simulink model "Btech_sys1"  (R2023b)
settings: Solver=VariableStepAuto  StartTime=0.0  StopTime=50  RelTol=1e-3
values from neighbouring files (symbols this model uses):
  Kd1 = x(1,3)    [fopid_pso.m]    (also in main_SHO_FOPID.m = Sea_horses(i,2); main_SHO_FOPTID.m = Sea_horses(i,2); main_SHO_PID.m = Sea_horses(i,2); pso.m)
  Kd2 = x(1,7)    [fopid_pso.m]    (also in main_SHO_FOPID.m = Sea_horses(i,5); main_SHO_FOPTID.m = Sea_horses(i,6); main_SHO_PID.m = Sea_horses(i,5); pso.m)
  Ki1 = x(1,2)    [fopid_pso.m]    (also in main_SHO_FOPID.m = Sea_horses(i,3); main_SHO_FOPTID.m = Sea_horses(i,3); main_SHO_PID.m = Sea_horses(i,3); pso.m)
  Ki2 = x(1,6)    [fopid_pso.m]    (also in main_SHO_FOPID.m = Sea_horses(i,6); main_SHO_FOPTID.m = Sea_horses(i,7); main_SHO_PID.m = Sea_horses(i,6); pso.m)
  Kp1 = x(1,1)    [fopid_pso.m]    (also in main_SHO_FOPID.m = Sea_horses(i,1); main_SHO_FOPTID.m = Sea_horses(i,1); main_SHO_PID.m = Sea_horses(i,1); pso.m)
  Kp2 = x(1,5)    [fopid_pso.m]    (also in main_SHO_FOPID.m = Sea_horses(i,4); main_SHO_FOPTID.m = Sea_horses(i,5); main_SHO_PID.m = Sea_horses(i,4); pso.m)
  Kt1 = Sea_horses(i,4)    [main_SHO_FOPTID.m]
  Kt2 = Sea_horses(i,8)    [main_SHO_FOPTID.m]
  N1 = Sea_horses(i,15)    [main_SHO_FOPTID.m]    (also in main_SHO_PID.m = Sea_horses(i,7); pso.m = x(1,4))
  N2 = Sea_horses(i,16)    [main_SHO_FOPTID.m]    (also in main_SHO_PID.m = Sea_horses(i,8); pso.m = x(1,8))
libraries: fod x10, slpidlib x2
settings Model: Creator=V.Abhijith  LastModifiedBy=V.Abhijith

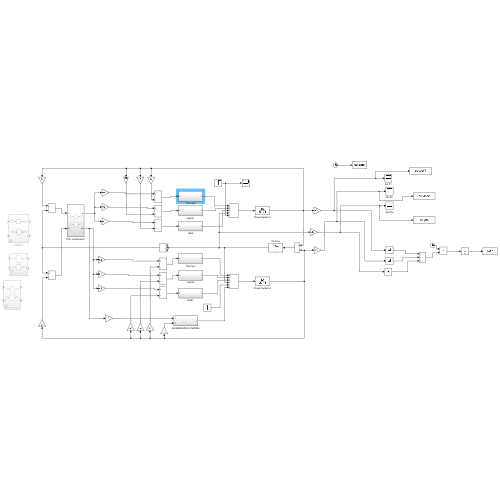
[thumbnail: Simulink's stored preview of the top-level diagram]
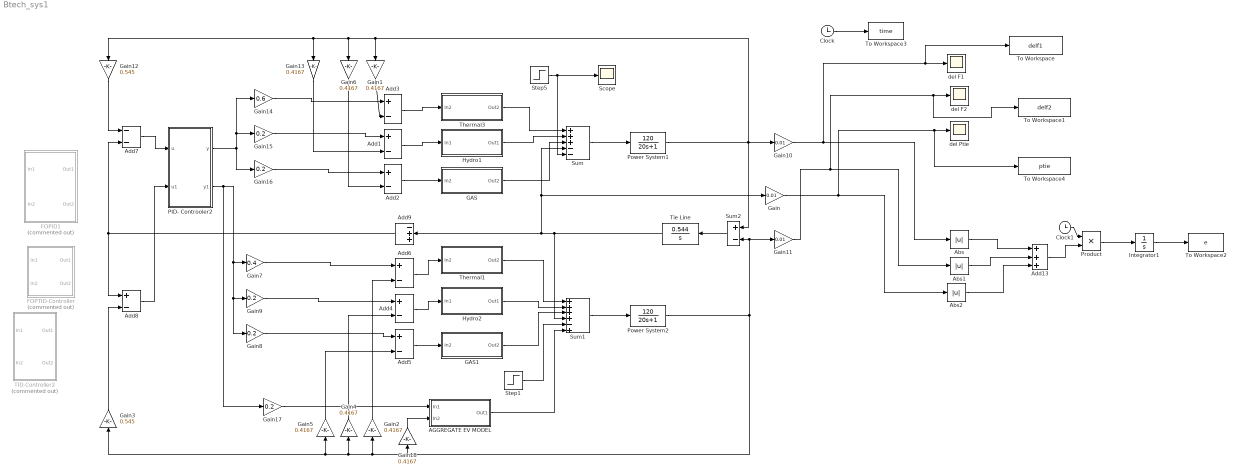
== system Btech_sys1 ==
  AGGREGATE EV MODEL : Subsystem
  Abs : Abs  SaturateOnIntegerOverflow=off
  Abs1 : Abs  SaturateOnIntegerOverflow=off
  Abs2 : Abs  SaturateOnIntegerOverflow=off
  Add{1..6,8} (7 alike) : Sum  Inputs=+-
  Add13 : Sum  Inputs=+++
  Add7 : Sum  Inputs=--
  Add9 : Sum  Inputs=-++
  Clock : Clock
  Clock1 : Clock
  FOPID1 : Subsystem  Commented=on
  FOPTID-Controller : Subsystem  Commented=on
  GAS : Subsystem
  GAS1 : Subsystem
  Gain : Gain  Gain=0.01
  Gain{1..2,4..6,13,18} (7 alike) : Gain  Gain=0.4167
  Gain10 : Gain  Gain=0.01
  Gain11 : Gain  Gain=0.01
  Gain12 : Gain  Gain=0.545
  Gain14 : Gain  Gain=0.6
  Gain{8..9,15..17} (5 alike) : Gain  Gain=0.2
  Gain3 : Gain  Gain=0.545
  Gain7 : Gain  Gain=0.4
  Hydro1 : Subsystem
  Hydro2 : Subsystem
  Integrator1 : Integrator
  PID- Controoler2 : Subsystem
  Power System1 : TransferFcn  Numerator=[120]  Denominator=[20 1]
  Power System2 : TransferFcn  Numerator=[120]  Denominator=[20 1]
  Product : Product
  Scope : Scope
  Step1 : Step  Time=0  After=0.03  SampleTime=0  ZeroCross=off
  Step5 : Step  Time=0  After=0.03  SampleTime=0  ZeroCross=off
  Sum : Sum  Inputs=+++--
  Sum1 : Sum  Inputs=++++-+
  Sum2 : Sum  Inputs=+-
  TID-Controller2 : Subsystem  Commented=on
  Thermal1 : Subsystem
  Thermal3 : Subsystem
  Tie Line : TransferFcn  Numerator=[0.544]  Denominator=[1 0]
  To Workspace : ToWorkspace  VariableName=delf1  SaveFormat=Timeseries  SampleTime=-1
  To Workspace1 : ToWorkspace  VariableName=delf2  SaveFormat=Timeseries  SampleTime=-1
  To Workspace2 : ToWorkspace  VariableName=e  SampleTime=-1
      settings: MaxDataPoints=1
  To Workspace3 : ToWorkspace  VariableName=time  SampleTime=-1
  To Workspace4 : ToWorkspace  VariableName=ptie  SaveFormat=Timeseries  SampleTime=-1
  del F1 : Scope
  del F2 : Scope
  del Ptie : Scope
  wires:
  Add8/1 -> PID- Controoler2/2(u1)
  Abs1/1 -> Add13/2
  Add4/1 -> Hydro2/1(In1)
  Step1/1 -> Sum1/5
  Tie Line/1 -> Add9/2, Gain/1, Sum/4, Sum1/4
  Abs2/1 -> Add13/3
  Add2/1 -> GAS/1(In2)
  Integrator1/1 -> To Workspace2/1
  Clock1/1 -> Product/1
  GAS1/1(Out2) -> Sum1/3
  PID- Controoler2/1(y) -> Gain16/1, Gain15/1, Gain14/1
  GAS/1(Out2) -> Sum/3
  Gain13/1 -> Add1/2
  Power System1/1 -> Gain10/1, Sum2/1, Gain12/1, Gain13/1, Gain6/1, Gain1/1
  Gain16/1 -> Add2/1
  Gain8/1 -> Add5/1
  Hydro2/1(Out1) -> Sum1/2
  Gain9/1 -> Add4/1
  Add1/1 -> Hydro1/1(In1)
  Hydro1/1(Out1) -> Sum/2
  Gain12/1 -> Add7/1
  Gain7/1 -> Add6/1
  Gain6/1 -> Add2/2
  Sum1/1 -> Power System2/1
  Sum/1 -> Power System1/1
  Gain5/1 -> Add5/2
  Add5/1 -> GAS1/1(In2)
  Sum2/1 -> Tie Line/1
  Thermal1/1(Out2) -> Sum1/1
  Product/1 -> Integrator1/1
  Gain3/1 -> Add8/2
  Power System2/1 -> Gain11/1, Sum2/2, Gain18/1, Gain3/1, Gain5/1, Gain4/1, Gain2/1
  Clock/1 -> To Workspace3/1
  Add9/1 -> Add8/1, Add7/2
  Step5/1 -> Sum/5, Scope/1
  Gain1/1 -> Add3/2
  Add6/1 -> Thermal1/1(In2)
  Gain4/1 -> Add4/2
  Abs/1 -> Add13/1
  Add7/1 -> PID- Controoler2/1(u)
  Gain2/1 -> Add6/2
  Gain15/1 -> Add1/1
  Gain14/1 -> Add3/1
  PID- Controoler2/2(y1) -> Gain17/1, Gain8/1, Gain9/1, Gain7/1
  Add13/1 -> Product/2
  Add3/1 -> Thermal3/1(In2)
  Thermal3/1(Out2) -> Sum/1
  AGGREGATE EV MODEL/1(Out1) -> Sum1/6
  Gain10/1 -> To Workspace/1, del F1/1, Abs/1
  Gain/1 -> To Workspace4/1, del Ptie/1, Abs2/1
  Gain11/1 -> To Workspace1/1, del F2/1, Abs1/1
  Gain17/1 -> AGGREGATE EV MODEL/1(In1)
  Gain18/1 -> AGGREGATE EV MODEL/2(In2)

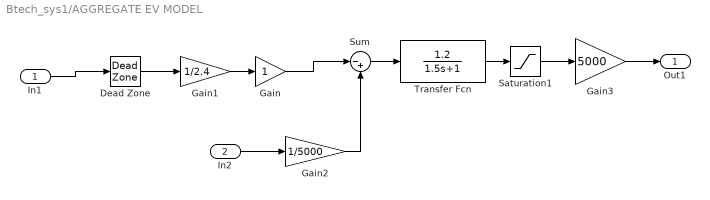
== system Btech_sys1/AGGREGATE EV MODEL ==
  In1 : Inport
  In2 : Inport  Port=2
  Dead Zone : DeadZone  LowerValue=-0.01  UpperValue=0.01
  Gain : Gain
  Gain1 : Gain  Gain=1/2.4
  Gain2 : Gain  Gain=1/5000
  Gain3 : Gain  Gain=5000
  Saturation1 : Saturate  UpperLimit=0.01  LowerLimit=-0.01
  Sum : Sum  Inputs=|-+
  Transfer Fcn : TransferFcn  Numerator=[1.2]  Denominator=[1.5 1]
  Out1 : Outport
  wires:
  Gain1/1 -> Gain/1
  Dead Zone/1 -> Gain1/1
  Sum/1 -> Transfer Fcn/1
  Gain/1 -> Sum/1
  Gain2/1 -> Sum/2
  In2/1 -> Gain2/1
  Transfer Fcn/1 -> Saturation1/1
  Saturation1/1 -> Gain3/1
  Gain3/1 -> Out1/1
  In1/1 -> Dead Zone/1

== system Btech_sys1/FOPID1 ==
  In1 : Inport
  In2 : Inport  Port=2
  Fractional PID controller1 : fod/Fractional PID controller  Kp=Kp2  Ki=Ki2  lambda=l2  Kd=Kd2  mic=m2  freqRange=[0.001, 1000]  N=5
      settings: SourceProductName=FOMCON Toolbox
  Fractional PID controller2 : fod/Fractional PID controller  Kp=Kp1  Ki=Ki1  lambda=l1  Kd=Kd1  mic=m1  freqRange=[0.001, 1000]  N=5
      settings: SourceProductName=FOMCON Toolbox
  Out1 : Outport
  Out2 : Outport  Port=2
  wires:
  In2/1 -> Fractional PID controller1/1
  Fractional PID controller2/1 -> Out1/1
  Fractional PID controller1/1 -> Out2/1
  In1/1 -> Fractional PID controller2/1

== system Btech_sys1/FOPTID-Controller ==
  In1 : Inport
  In2 : Inport  Port=2
  FOPTID : Subsystem
  FOPTID1 : Subsystem
  Out1 : Outport
  Out2 : Outport  Port=2
  wires:
  In1/1 -> FOPTID/1(In1)
  In2/1 -> FOPTID1/1(In1)
  FOPTID1/1(Out1) -> Out2/1
  FOPTID/1(Out1) -> Out1/1

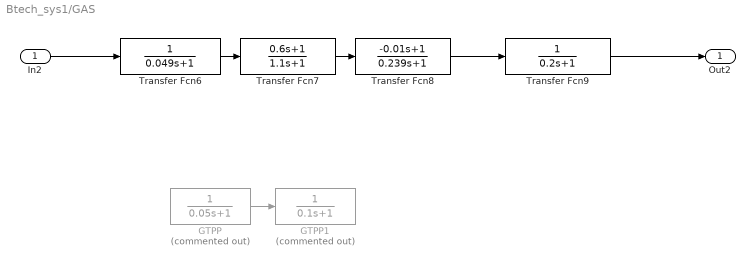
== system Btech_sys1/GAS ==
  In2 : Inport
  GTPP : TransferFcn  Commented=on  Denominator=[0.05 1]
  GTPP1 : TransferFcn  Commented=on  Denominator=[0.1 1]
  Transfer Fcn6 : TransferFcn  Denominator=[0.049 1]
  Transfer Fcn7 : TransferFcn  Numerator=[0.6 1]  Denominator=[1.1 1]
  Transfer Fcn8 : TransferFcn  Numerator=[-0.01 1]  Denominator=[0.239 1]
  Transfer Fcn9 : TransferFcn  Denominator=[0.2 1]
  Out2 : Outport
  wires:
  GTPP/1 -> GTPP1/1
  In2/1 -> Transfer Fcn6/1
  Transfer Fcn7/1 -> Transfer Fcn8/1
  Transfer Fcn6/1 -> Transfer Fcn7/1
  Transfer Fcn8/1 -> Transfer Fcn9/1
  Transfer Fcn9/1 -> Out2/1

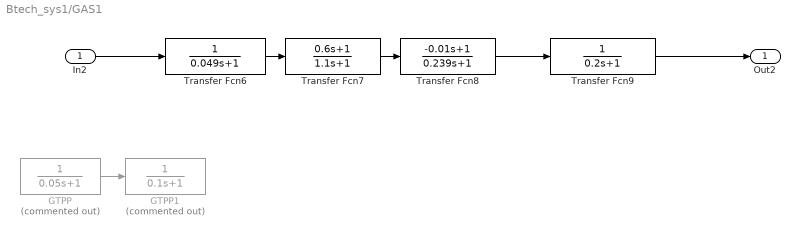
== system Btech_sys1/GAS1 ==
  In2 : Inport
  GTPP : TransferFcn  Commented=on  Denominator=[0.05 1]
  GTPP1 : TransferFcn  Commented=on  Denominator=[0.1 1]
  Transfer Fcn6 : TransferFcn  Denominator=[0.049 1]
  Transfer Fcn7 : TransferFcn  Numerator=[0.6 1]  Denominator=[1.1 1]
  Transfer Fcn8 : TransferFcn  Numerator=[-0.01 1]  Denominator=[0.239 1]
  Transfer Fcn9 : TransferFcn  Denominator=[0.2 1]
  Out2 : Outport
  wires:
  GTPP/1 -> GTPP1/1
  In2/1 -> Transfer Fcn6/1
  Transfer Fcn7/1 -> Transfer Fcn8/1
  Transfer Fcn6/1 -> Transfer Fcn7/1
  Transfer Fcn8/1 -> Transfer Fcn9/1
  Transfer Fcn9/1 -> Out2/1

== system Btech_sys1/Hydro1 ==
  In1 : Inport
  Transfer Fcn : TransferFcn  Denominator=[0.2 1]
  Transfer Fcn1 : TransferFcn  Numerator=[-1 1]  Denominator=[0.5 1]
  Transfer Fcn2 : TransferFcn  Numerator=[5 1]  Denominator=[28.75 1]
  Out1 : Outport
  wires:
  In1/1 -> Transfer Fcn/1
  Transfer Fcn/1 -> Transfer Fcn2/1
  Transfer Fcn2/1 -> Transfer Fcn1/1
  Transfer Fcn1/1 -> Out1/1

== system Btech_sys1/Hydro2 ==
  In1 : Inport
  Transfer Fcn : TransferFcn  Denominator=[0.2 1]
  Transfer Fcn1 : TransferFcn  Numerator=[-1 1]  Denominator=[0.5 1]
  Transfer Fcn2 : TransferFcn  Numerator=[5 1]  Denominator=[28.75 1]
  Out1 : Outport
  wires:
  In1/1 -> Transfer Fcn/1
  Transfer Fcn/1 -> Transfer Fcn2/1
  Transfer Fcn2/1 -> Transfer Fcn1/1
  Transfer Fcn1/1 -> Out1/1

== system Btech_sys1/PID- Controoler2 ==
  u : Inport
  u1 : Inport  Port=2
  PID Controller : slpidlib/PID Controller  Controller=PID  Form=Parallel  TimeDomain=Continuous-time  UseExternalTs=off  SampleTime=-1  IntegratorMethod=Forward Euler  FilterMethod=Forward Euler  ControllerParametersSource=internal  P=Kp1  I=Ki1  UseKiTs=off  D=Kd1  N=N1  UseFilter=on  TunerSelectOption=Transfer Function Based (PID Tuner App)  InitialConditionSource=internal  InitialConditionForIntegrator=0  InitialConditionForFilter=0  DifferentiatorICPrevScaledInput=0  ExternalReset=none  TrackingMode=off  Kt=1  LimitOutput=off  SatLimitsSource=internal  UpperSaturationLimit=inf  LowerSaturationLimit=-inf  LinearizeAsGain=on  AntiWindupMode=none  Kb=1  LimitIntegrator=off  UpperIntegratorSaturationLimit=inf  LowerIntegratorSaturationLimit=-inf  POutMin=[]  POutMax=[]  IOutMin=[]  IOutMax=[]  DOutMin=[]  DOutMax=[]  NOutMin=[]  NOutMax=[]  SumOutMin=[]  SumOutMax=[]  SaturationOutMin=[]  SaturationOutMax=[]  PParamMin=[]  PParamMax=[]  IParamMin=[]  IParamMax=[]  DParamMin=[]  DParamMax=[]  NParamMin=[]  NParamMax=[]  KbParamMin=[]  KbParamMax=[]  KtParamMin=[]  KtParamMax=[]  KbOutMin=[]  KbOutMax=[]  KtOutMin=[]  KtOutMax=[]  IntegratorOutMin=[]  IntegratorOutMax=[]  FilterOutMin=[]  FilterOutMax=[]  SumI1OutMin=[]  SumI1OutMax=[]  SumI2OutMin=[]  SumI2OutMax=[]  SumI3OutMin=[]  SumI3OutMax=[]  SumI4OutMin=[]  SumI4OutMax=[]  SumDOutMin=[]  SumDOutMax=[]  DifferentiatorOutMin=[]  DifferentiatorOutMax=[]  FilterDiffOutCoefMin=[]  FilterDiffOutCoefMax=[]  ReciprocalOutMin=[]  ReciprocalOutMax=[]  SumDenOutMin=[]  SumDenOutMax=[]  SumNumOutMin=[]  SumNumOutMax=[]  DivideOutMin=[]  DivideOutMax=[]  UdiffTsProdOutMin=[]  UdiffTsProdOutMax=[]  NTsProdOutMin=[]  NTsProdOutMax=[]  UintegralTsProdOutMin=[]  UintegralTsProdOutMax=[]  UngainTsProdOutMin=[]  UngainTsProdOutMax=[]  ClampingZeroOutDataTypeStr=Inherit: Inherit via back propagation  ClampingZeroOutMin=[]  ClampingZeroOutMax=[]  FilterDenConstantOutDataTypeStr=Inherit: Inherit via back propagation  FilterDenConstantOutMin=[]  FilterDenConstantOutMax=[]  PCopyOutDataTypeStr=Inherit: Inherit via back propagation  PCopyOutMin=[]  PCopyOutMax=[]  NCopyOutDataTypeStr=Inherit: Inherit via back propagation  NCopyOutMin=[]  NCopyOutMax=[]  IntegratorContinuousStateAttributes=''  IntegratorStateMustResolveToSignalObject=off  IntegratorRTWStateStorageClass=Auto  FilterContinuousStateAttributes=''  FilterStateMustResolveToSignalObject=off  FilterRTWStateStorageClass=Auto  ParallelPVariant=InternalParameters  IdealPVariant=Disabled  IVariant=InternalParameters  DVariant=InternalParameters  IntegratorVariant=Continuous  SatVariant=Disabled  AWVariant=Passthrough  PCopyVariant=Disabled  TRVariant=Disabled  FdbkBlocksVariant=Forward  IdealPFdbkVariant=Disabled  SatFdbkVariant=Disabled  DerivativeFilterVariant=ContFilter  NVariant=InternalParameters  NCopyVariant=Disabled  FilterICVariant=InternalICsFilter  IntegratorICVariant=InternalICs  ExternalResetVariant=Disabled  TRSumVariant=Passthrough  SumFdbkVariant=Disabled  SumVariant=Sum_PID  TsampFilterVariant=InternalTs  TsampNgainVariant=Passthrough  TsampIntegralVariant=Disabled_SignalSpec  ExternalSaturationOutDataTypeStr=Inherit: Same as second input
  PID Controller1 : slpidlib/PID Controller  Controller=PID  Form=Parallel  TimeDomain=Continuous-time  UseExternalTs=off  SampleTime=-1  IntegratorMethod=Forward Euler  FilterMethod=Forward Euler  ControllerParametersSource=internal  P=Kp2  I=Ki2  UseKiTs=off  D=Kd2  N=N2  UseFilter=on  TunerSelectOption=Transfer Function Based (PID Tuner App)  InitialConditionSource=internal  InitialConditionForIntegrator=0  InitialConditionForFilter=0  DifferentiatorICPrevScaledInput=0  ExternalReset=none  TrackingMode=off  Kt=1  LimitOutput=off  SatLimitsSource=internal  UpperSaturationLimit=inf  LowerSaturationLimit=-inf  LinearizeAsGain=on  AntiWindupMode=none  Kb=1  LimitIntegrator=off  UpperIntegratorSaturationLimit=inf  LowerIntegratorSaturationLimit=-inf  POutMin=[]  POutMax=[]  IOutMin=[]  IOutMax=[]  DOutMin=[]  DOutMax=[]  NOutMin=[]  NOutMax=[]  SumOutMin=[]  SumOutMax=[]  SaturationOutMin=[]  SaturationOutMax=[]  PParamMin=[]  PParamMax=[]  IParamMin=[]  IParamMax=[]  DParamMin=[]  DParamMax=[]  NParamMin=[]  NParamMax=[]  KbParamMin=[]  KbParamMax=[]  KtParamMin=[]  KtParamMax=[]  KbOutMin=[]  KbOutMax=[]  KtOutMin=[]  KtOutMax=[]  IntegratorOutMin=[]  IntegratorOutMax=[]  FilterOutMin=[]  FilterOutMax=[]  SumI1OutMin=[]  SumI1OutMax=[]  SumI2OutMin=[]  SumI2OutMax=[]  SumI3OutMin=[]  SumI3OutMax=[]  SumI4OutMin=[]  SumI4OutMax=[]  SumDOutMin=[]  SumDOutMax=[]  DifferentiatorOutMin=[]  DifferentiatorOutMax=[]  FilterDiffOutCoefMin=[]  FilterDiffOutCoefMax=[]  ReciprocalOutMin=[]  ReciprocalOutMax=[]  SumDenOutMin=[]  SumDenOutMax=[]  SumNumOutMin=[]  SumNumOutMax=[]  DivideOutMin=[]  DivideOutMax=[]  UdiffTsProdOutMin=[]  UdiffTsProdOutMax=[]  NTsProdOutMin=[]  NTsProdOutMax=[]  UintegralTsProdOutMin=[]  UintegralTsProdOutMax=[]  UngainTsProdOutMin=[]  UngainTsProdOutMax=[]  ClampingZeroOutDataTypeStr=Inherit: Inherit via back propagation  ClampingZeroOutMin=[]  ClampingZeroOutMax=[]  FilterDenConstantOutDataTypeStr=Inherit: Inherit via back propagation  FilterDenConstantOutMin=[]  FilterDenConstantOutMax=[]  PCopyOutDataTypeStr=Inherit: Inherit via back propagation  PCopyOutMin=[]  PCopyOutMax=[]  NCopyOutDataTypeStr=Inherit: Inherit via back propagation  NCopyOutMin=[]  NCopyOutMax=[]  IntegratorContinuousStateAttributes=''  IntegratorStateMustResolveToSignalObject=off  IntegratorRTWStateStorageClass=Auto  FilterContinuousStateAttributes=''  FilterStateMustResolveToSignalObject=off  FilterRTWStateStorageClass=Auto  ParallelPVariant=InternalParameters  IdealPVariant=Disabled  IVariant=InternalParameters  DVariant=InternalParameters  IntegratorVariant=Continuous  SatVariant=Disabled  AWVariant=Passthrough  PCopyVariant=Disabled  TRVariant=Disabled  FdbkBlocksVariant=Forward  IdealPFdbkVariant=Disabled  SatFdbkVariant=Disabled  DerivativeFilterVariant=ContFilter  NVariant=InternalParameters  NCopyVariant=Disabled  FilterICVariant=InternalICsFilter  IntegratorICVariant=InternalICs  ExternalResetVariant=Disabled  TRSumVariant=Passthrough  SumFdbkVariant=Disabled  SumVariant=Sum_PID  TsampFilterVariant=InternalTs  TsampNgainVariant=Passthrough  TsampIntegralVariant=Disabled_SignalSpec  ExternalSaturationOutDataTypeStr=Inherit: Same as second input
  y : Outport
  y1 : Outport  Port=2
  wires:
  PID Controller1/1 -> y1/1
  PID Controller/1 -> y/1
  u/1 -> PID Controller/1
  u1/1 -> PID Controller1/1

== system Btech_sys1/TID-Controller2 ==
  In1 : Inport
  In2 : Inport  Port=2
  TID : Subsystem
  TID1 : Subsystem
  Out1 : Outport
  Out2 : Outport  Port=2
  wires:
  TID/1(Out1) -> Out1/1
  In1/1 -> TID/1(In1)
  In2/1 -> TID1/1(In1)
  TID1/1(Out1) -> Out2/1

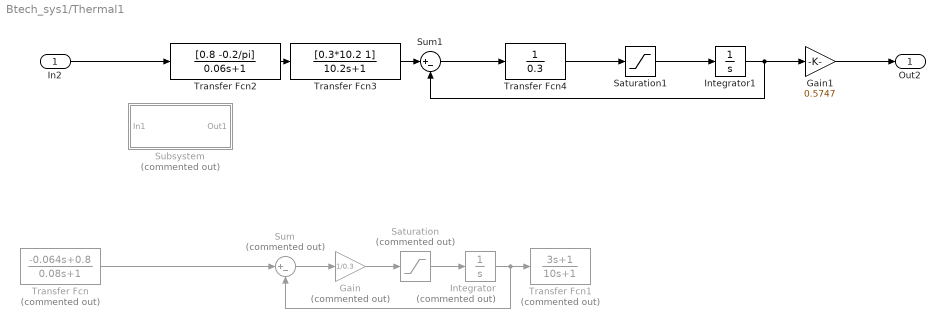
== system Btech_sys1/Thermal1 ==
  In2 : Inport
  Gain : Gain  Commented=on  Gain=1/0.3
  Gain1 : Gain  Gain=0.5747
  Integrator : Integrator  Commented=on
  Integrator1 : Integrator
  Saturation : Saturate  Commented=on  UpperLimit=0.0005  LowerLimit=-0.0005
  Saturation1 : Saturate  UpperLimit=0.0017  LowerLimit=-0.0017  ZeroCross=off
  Subsystem : Subsystem  Commented=on
  Sum : Sum  Commented=on  Inputs=|+-
  Sum1 : Sum  Inputs=|+-
  Transfer Fcn : TransferFcn  Commented=on  Numerator=[-0.064 0.8]  Denominator=[0.08 1]
  Transfer Fcn1 : TransferFcn  Commented=on  Numerator=[3 1]  Denominator=[10 1]
  Transfer Fcn2 : TransferFcn  Numerator=[0.8 -0.2/pi]  Denominator=[0.06 1]
  Transfer Fcn3 : TransferFcn  Numerator=[0.3*10.2 1]  Denominator=[10.2 1]
  Transfer Fcn4 : TransferFcn  Denominator=[0.3]
  Out2 : Outport
  wires:
  Gain/1 -> Saturation/1
  Transfer Fcn/1 -> Sum/1
  Sum/1 -> Gain/1
  Saturation/1 -> Integrator/1
  Integrator/1 -> Sum/2, Transfer Fcn1/1
  In2/1 -> Transfer Fcn2/1
  Transfer Fcn3/1 -> Sum1/1
  Integrator1/1 -> Sum1/2, Gain1/1
  Transfer Fcn4/1 -> Saturation1/1
  Transfer Fcn2/1 -> Transfer Fcn3/1
  Sum1/1 -> Transfer Fcn4/1
  Gain1/1 -> Out2/1
  Saturation1/1 -> Integrator1/1

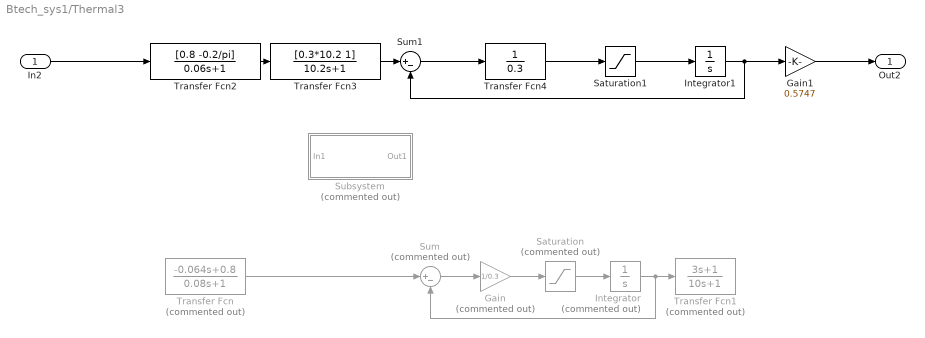
== system Btech_sys1/Thermal3 ==
  In2 : Inport
  Gain : Gain  Commented=on  Gain=1/0.3
  Gain1 : Gain  Gain=0.5747
  Integrator : Integrator  Commented=on
  Integrator1 : Integrator
  Saturation : Saturate  Commented=on  UpperLimit=0.0005  LowerLimit=-0.0005
  Saturation1 : Saturate  UpperLimit=0.0017  LowerLimit=-0.0017  ZeroCross=off
  Subsystem : Subsystem  Commented=on
  Sum : Sum  Commented=on  Inputs=|+-
  Sum1 : Sum  Inputs=|+-
  Transfer Fcn : TransferFcn  Commented=on  Numerator=[-0.064 0.8]  Denominator=[0.08 1]
  Transfer Fcn1 : TransferFcn  Commented=on  Numerator=[3 1]  Denominator=[10 1]
  Transfer Fcn2 : TransferFcn  Numerator=[0.8 -0.2/pi]  Denominator=[0.06 1]
  Transfer Fcn3 : TransferFcn  Numerator=[0.3*10.2 1]  Denominator=[10.2 1]
  Transfer Fcn4 : TransferFcn  Denominator=[0.3]
  Out2 : Outport
  wires:
  Gain/1 -> Saturation/1
  Transfer Fcn/1 -> Sum/1
  Sum/1 -> Gain/1
  Saturation/1 -> Integrator/1
  Integrator/1 -> Sum/2, Transfer Fcn1/1
  In2/1 -> Transfer Fcn2/1
  Transfer Fcn3/1 -> Sum1/1
  Integrator1/1 -> Sum1/2, Gain1/1
  Transfer Fcn4/1 -> Saturation1/1
  Transfer Fcn2/1 -> Transfer Fcn3/1
  Sum1/1 -> Transfer Fcn4/1
  Gain1/1 -> Out2/1
  Saturation1/1 -> Integrator1/1

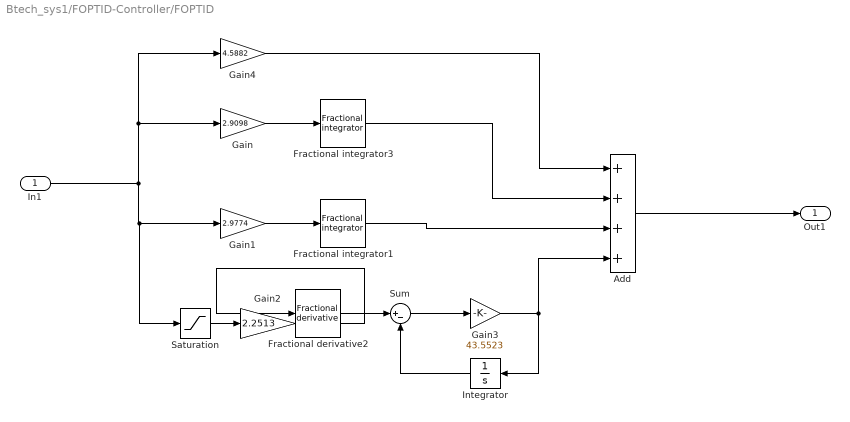
== system Btech_sys1/FOPTID-Controller/FOPTID ==
  In1 : Inport
  Add : Sum  Inputs=++++
  Fractional derivative2 : fod/Fractional derivative  gam=0.4641  ww=[0.001; 1000]  n=5  nFod=off
      settings: SourceProductName=FOMCON Toolbox
  Fractional integrator1 : fod/Fractional integrator  gam=0.9431  ww=[0.001; 1000]  n=5  nFod=off
      settings: SourceProductName=FOMCON Toolbox
  Fractional integrator3 : fod/Fractional integrator  gam=0.6355  ww=[0.001; 1000]  n=5  nFod=on
      settings: SourceProductName=FOMCON Toolbox
  Gain : Gain  Gain=2.9098
  Gain1 : Gain  Gain=2.9774
  Gain2 : Gain  Gain=2.2513
  Gain3 : Gain  Gain=43.5523
  Gain4 : Gain  Gain=4.5882
  Integrator : Integrator
  Saturation : Saturate  UpperLimit=100000  LowerLimit=-100000
  Sum : Sum  Inputs=|+-
  Out1 : Outport
  wires:
  Gain/1 -> Fractional integrator3/1
  In1/1 -> Saturation/1, Gain1/1, Gain/1, Gain4/1
  Integrator/1 -> Sum/2
  Fractional derivative2/1 -> Sum/1
  Gain3/1 -> Integrator/1, Add/4
  Gain2/1 -> Fractional derivative2/1
  Sum/1 -> Gain3/1
  Gain1/1 -> Fractional integrator1/1
  Add/1 -> Out1/1
  Fractional integrator3/1 -> Add/2
  Gain4/1 -> Add/1
  Fractional integrator1/1 -> Add/3
  Saturation/1 -> Gain2/1

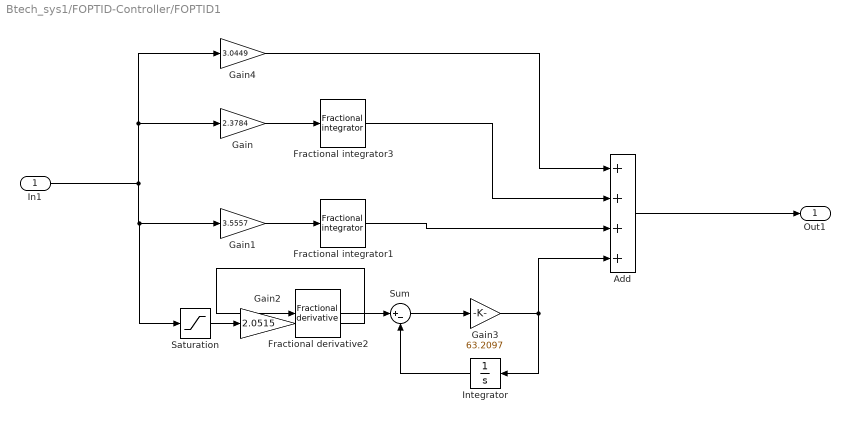
== system Btech_sys1/FOPTID-Controller/FOPTID1 ==
  In1 : Inport
  Add : Sum  Inputs=++++
  Fractional derivative2 : fod/Fractional derivative  gam=0.3584  ww=[0.001; 1000]  n=5  nFod=off
      settings: SourceProductName=FOMCON Toolbox
  Fractional integrator1 : fod/Fractional integrator  gam=0.8302  ww=[0.001; 1000]  n=5  nFod=off
      settings: SourceProductName=FOMCON Toolbox
  Fractional integrator3 : fod/Fractional integrator  gam=0.6355  ww=[0.001; 1000]  n=5  nFod=on
      settings: SourceProductName=FOMCON Toolbox
  Gain : Gain  Gain=2.3784
  Gain1 : Gain  Gain=3.5557
  Gain2 : Gain  Gain=2.0515
  Gain3 : Gain  Gain=63.2097
  Gain4 : Gain  Gain=3.0449
  Integrator : Integrator
  Saturation : Saturate  UpperLimit=100000  LowerLimit=-100000
  Sum : Sum  Inputs=|+-
  Out1 : Outport
  wires:
  Saturation/1 -> Gain2/1
  Fractional integrator1/1 -> Add/3
  Gain4/1 -> Add/1
  Fractional integrator3/1 -> Add/2
  Add/1 -> Out1/1
  Gain1/1 -> Fractional integrator1/1
  Sum/1 -> Gain3/1
  Gain2/1 -> Fractional derivative2/1
  Gain3/1 -> Add/4, Integrator/1
  Fractional derivative2/1 -> Sum/1
  Integrator/1 -> Sum/2
  In1/1 -> Gain4/1, Gain/1, Gain1/1, Saturation/1
  Gain/1 -> Fractional integrator3/1

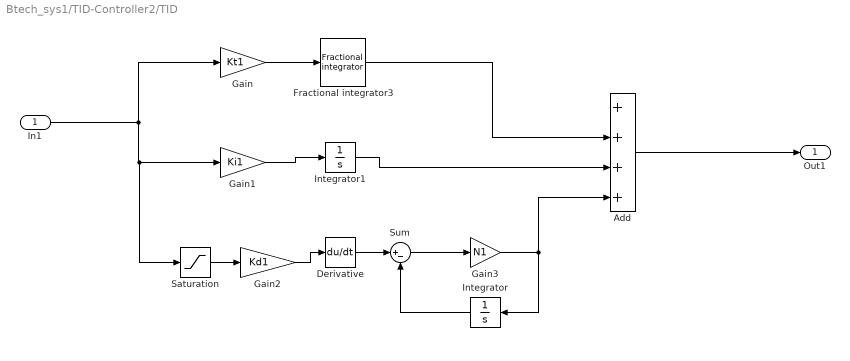
== system Btech_sys1/TID-Controller2/TID ==
  In1 : Inport
  Add : Sum  Inputs=++++
  Derivative : Derivative
  Fractional integrator3 : fod/Fractional integrator  gam=n1  ww=[0.001; 1000]  n=5  nFod=on
      settings: SourceProductName=FOMCON Toolbox
  Gain : Gain  Gain=Kt1
  Gain1 : Gain  Gain=Ki1
  Gain2 : Gain  Gain=Kd1
  Gain3 : Gain  Gain=N1
  Integrator : Integrator
  Integrator1 : Integrator
  Saturation : Saturate  UpperLimit=100000  LowerLimit=-100000
  Sum : Sum  Inputs=|+-
  Out1 : Outport
  wires:
  Gain/1 -> Fractional integrator3/1
  In1/1 -> Saturation/1, Gain1/1, Gain/1
  Integrator/1 -> Sum/2
  Derivative/1 -> Sum/1
  Gain3/1 -> Integrator/1, Add/4
  Sum/1 -> Gain3/1
  Add/1 -> Out1/1
  Fractional integrator3/1 -> Add/2
  Integrator1/1 -> Add/3
  Saturation/1 -> Gain2/1
  Gain1/1 -> Integrator1/1
  Gain2/1 -> Derivative/1

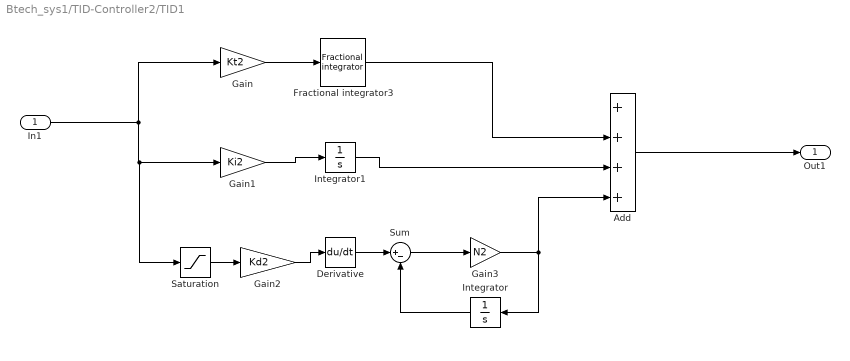
== system Btech_sys1/TID-Controller2/TID1 ==
  In1 : Inport
  Add : Sum  Inputs=++++
  Derivative : Derivative
  Fractional integrator3 : fod/Fractional integrator  gam=n2  ww=[0.001; 1000]  n=5  nFod=on
      settings: SourceProductName=FOMCON Toolbox
  Gain : Gain  Gain=Kt2
  Gain1 : Gain  Gain=Ki2
  Gain2 : Gain  Gain=Kd2
  Gain3 : Gain  Gain=N2
  Integrator : Integrator
  Integrator1 : Integrator
  Saturation : Saturate  UpperLimit=100000  LowerLimit=-100000
  Sum : Sum  Inputs=|+-
  Out1 : Outport
  wires:
  Gain/1 -> Fractional integrator3/1
  In1/1 -> Saturation/1, Gain1/1, Gain/1
  Integrator/1 -> Sum/2
  Derivative/1 -> Sum/1
  Gain3/1 -> Integrator/1, Add/4
  Sum/1 -> Gain3/1
  Add/1 -> Out1/1
  Fractional integrator3/1 -> Add/2
  Integrator1/1 -> Add/3
  Saturation/1 -> Gain2/1
  Gain1/1 -> Integrator1/1
  Gain2/1 -> Derivative/1

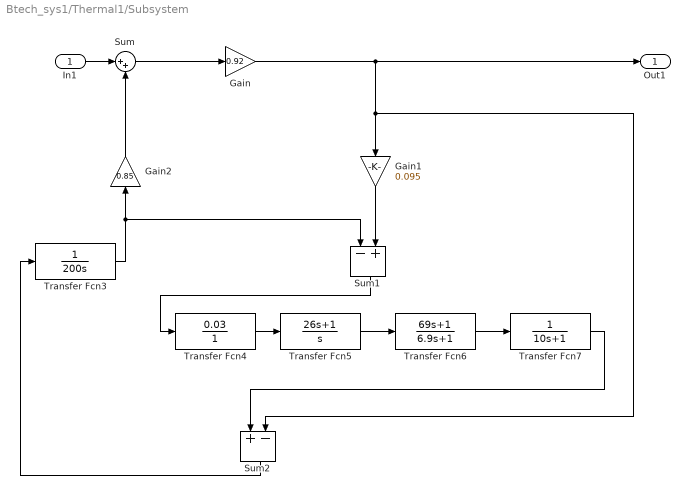
== system Btech_sys1/Thermal1/Subsystem ==
  In1 : Inport
  Gain : Gain  Gain=0.92
  Gain1 : Gain  Gain=0.095
  Gain2 : Gain  Gain=0.85
  Sum : Sum  Inputs=|++
  Sum1 : Sum  Inputs=-+
  Sum2 : Sum  Inputs=+-
  Transfer Fcn3 : TransferFcn  Denominator=[200 0]
  Transfer Fcn4 : TransferFcn  Numerator=[0.03]  Denominator=[0 1]
  Transfer Fcn5 : TransferFcn  Numerator=[26 1]  Denominator=[1 0]
  Transfer Fcn6 : TransferFcn  Numerator=[69 1]  Denominator=[6.9 1]
  Transfer Fcn7 : TransferFcn  Denominator=[10 1]
  Out1 : Outport
  wires:
  In1/1 -> Sum/1
  Sum/1 -> Gain/1
  Gain/1 -> Out1/1, Sum2/2, Gain1/1
  Gain1/1 -> Sum1/2
  Gain2/1 -> Sum/2
  Transfer Fcn3/1 -> Sum1/1, Gain2/1
  Transfer Fcn5/1 -> Transfer Fcn6/1
  Transfer Fcn4/1 -> Transfer Fcn5/1
  Sum1/1 -> Transfer Fcn4/1
  Transfer Fcn6/1 -> Transfer Fcn7/1
  Transfer Fcn7/1 -> Sum2/1
  Sum2/1 -> Transfer Fcn3/1

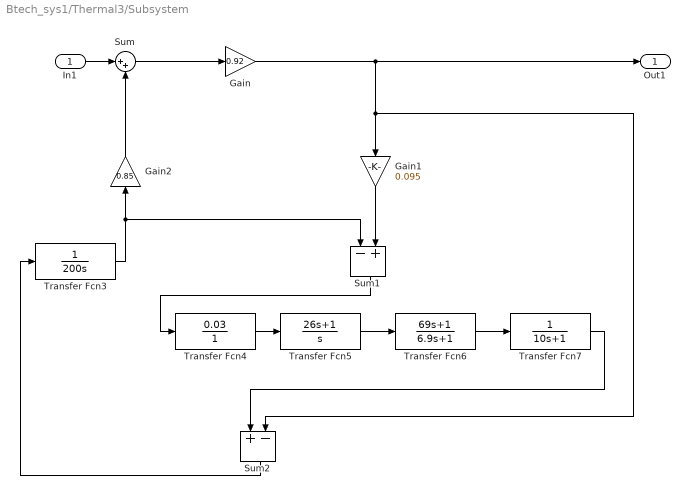
== system Btech_sys1/Thermal3/Subsystem ==
  In1 : Inport
  Gain : Gain  Gain=0.92
  Gain1 : Gain  Gain=0.095
  Gain2 : Gain  Gain=0.85
  Sum : Sum  Inputs=|++
  Sum1 : Sum  Inputs=-+
  Sum2 : Sum  Inputs=+-
  Transfer Fcn3 : TransferFcn  Denominator=[200 0]
  Transfer Fcn4 : TransferFcn  Numerator=[0.03]  Denominator=[0 1]
  Transfer Fcn5 : TransferFcn  Numerator=[26 1]  Denominator=[1 0]
  Transfer Fcn6 : TransferFcn  Numerator=[69 1]  Denominator=[6.9 1]
  Transfer Fcn7 : TransferFcn  Denominator=[10 1]
  Out1 : Outport
  wires:
  In1/1 -> Sum/1
  Sum/1 -> Gain/1
  Gain/1 -> Out1/1, Sum2/2, Gain1/1
  Gain1/1 -> Sum1/2
  Gain2/1 -> Sum/2
  Transfer Fcn3/1 -> Sum1/1, Gain2/1
  Transfer Fcn5/1 -> Transfer Fcn6/1
  Transfer Fcn4/1 -> Transfer Fcn5/1
  Sum1/1 -> Transfer Fcn4/1
  Transfer Fcn6/1 -> Transfer Fcn7/1
  Transfer Fcn7/1 -> Sum2/1
  Sum2/1 -> Transfer Fcn3/1
